simulink library "groundStation001_cl"  (R2018b)
settings: Solver=VariableStepAuto  StartTime=0.0  StopTime=10.0  RelTol=1e-3
undefined symbols (not defined in the file): CB2CMVec, flow, gndStnMmtArms, grav, inertiaMatrix, m, tetherLengths
libraries: thrAttachPtKinematics_ul x3, tethersMoment_cl x2, vrlib x1, eulAng2RotMat_ul x1, liftingBodyTension x1, circulationForce_ul x1, sixDoFDynamics_ul x1, tethers_cl x1, variableBuoyancy_ul x1
settings Model: Creator=Erin B  LastModifiedBy=mcobb

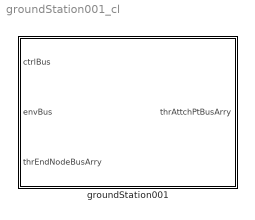
== system groundStation001_cl ==
  groundStation001 : Subsystem  mask{data=1, moments=0}
      mask prompts: data "Input lifting body forces or previously calculated lifting body forces? (0= input, 1 = previously calculated)"; moments "Calculate moments? (1 = yes, 0 = no)"

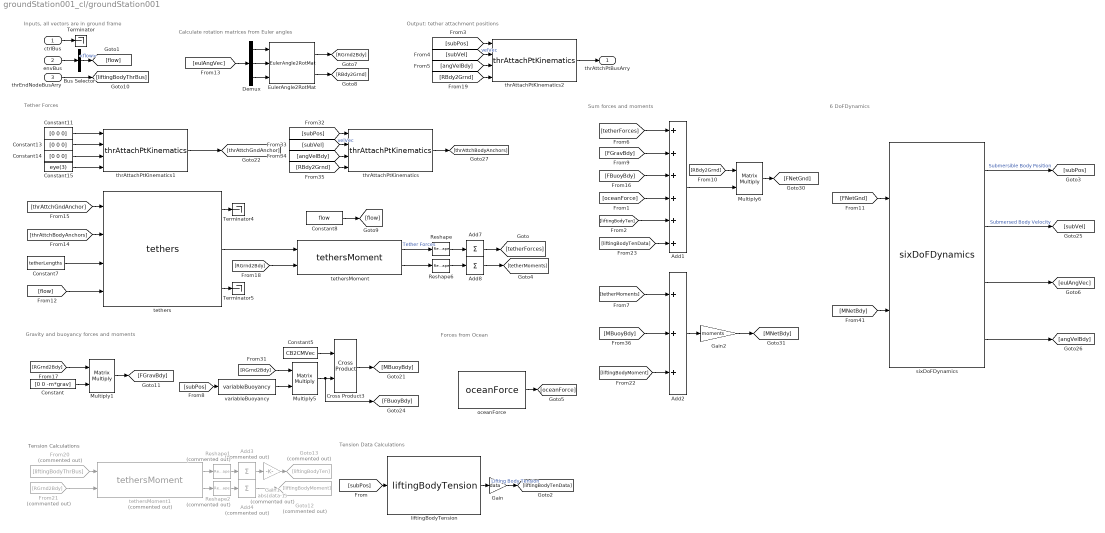
== system groundStation001_cl/groundStation001 ==
  note: Tension Calculations
  note: Tension Data Calculations
  note: Output: tether attachment positions
  note: Tether Forces
  note: Inputs, all vectors are in ground frame
  note: Calculate rotation matrices from Euler angles
  note: Sum forces and moments
  note: Gravity and buoyancy forces and moments
  note: 6 DoFDynamics
  note: Forces from Ocean
  ctrlBus : Inport  OutDataTypeStr=Bus: ctrlBus
  envBus : Inport  Port=2  OutDataTypeStr=Bus: envBus
  thrEndNodeBusArry : Inport  Port=3
  Add1 : Sum  Inputs=++++++
  Add2 : Sum  Inputs=+++
  Add3 : Sum  Commented=on  Inputs=+  CollapseMode=Specified dimension  CollapseDim=2
  Add4 : Sum  Commented=on  Inputs=+  CollapseMode=Specified dimension  CollapseDim=2
  Add7 : Sum  Inputs=+  CollapseMode=Specified dimension  CollapseDim=2
  Add8 : Sum  Inputs=+  CollapseMode=Specified dimension  CollapseDim=2
  Bus Selector : BusSelector  OutputSignals=flow
  Constant : Constant  Value=[0 0 -m*grav]
  Constant11 : Constant  Value=[0 0 0]
  Constant13 : Constant  Value=[0 0 0]
  Constant14 : Constant  Value=[0 0 0]
  Constant15 : Constant  Value=eye(3)
  Constant5 : Constant  Value=CB2CMVec
  Constant7 : Constant  Value=tetherLengths
  Constant8 : Constant  Value=flow
  Cross Product3 : vrlib/Utilities/Cross Product
      settings: SourceProductBaseCode=VR
  Demux : Demux  Outputs=3
  EulerAngle2RotMat : eulAng2RotMat_ul/EulerAngle2RotMat  SystemSampleTime=-1
  From20 : From  Commented=on  GotoTag=liftingBodyThrBus
  From21 : From  Commented=on  GotoTag=RGrnd2Bdy
  Gain : Gain  Gain=data
  Gain1 : Gain  Commented=on  Gain=abs(data-1)
  Gain2 : Gain  Gain=moments
  Goto12 : Goto  Commented=on  GotoTag=liftingBodyMoment
  Goto13 : Goto  Commented=on  GotoTag=liftingBodyTen
  Multiply1 : Product  Multiplication=Matrix(*)
  Multiply5 : Product  Multiplication=Matrix(*)
  Multiply6 : Product  Multiplication=Matrix(*)
  Reshape : Reshape  OutputDimensionality=Customize  OutputDimensions=[3 numel(gndStnMmtArms)]
  Reshape1 : Reshape  Commented=on  OutputDimensionality=Customize  OutputDimensions=[3 numel(gndStnMmtArms)]
  Reshape2 : Reshape  Commented=on  OutputDimensionality=Customize  OutputDimensions=[3 numel(gndStnMmtArms)]
  Reshape6 : Reshape  OutputDimensionality=Customize  OutputDimensions=[3 numel(gndStnMmtArms)]
  Terminator : Terminator
  Terminator4 : Terminator
  Terminator5 : Terminator
  liftingBodyTension : liftingBodyTension/liftingBodyTension  pos=position  mag=mag
  oceanForce : circulationForce_ul/oceanForce  SystemSampleTime=-1
  sixDoFDynamics : sixDoFDynamics_ul/sixDoFDynamics  M=mass  initPos=initPos  initVel=initVel  J=inertiaMatrix  initEulAngs=initEulerAngles  initAngVel=initAngVel
  tethers : tethers_cl/tethers   SystemSampleTime=-1
      link override VariantSubsystem: LabelModeActiveChoice=VSS_twoNodeTether
  tethersMoment : tethersMoment_cl/tethersMoment  arms=arms
  tethersMoment1 : tethersMoment_cl/tethersMoment  Commented=on  arms=arms
  thrAttachPtKinematics : thrAttachPtKinematics_ul/thrAttachPtKinematics  atchPts=bodyMmtArms
  thrAttachPtKinematics1 : thrAttachPtKinematics_ul/thrAttachPtKinematics  atchPts=gndStnMmtArms
  thrAttachPtKinematics2 : thrAttachPtKinematics_ul/thrAttachPtKinematics  atchPts=liftingBodyThrAttch
  variableBuoyancy : variableBuoyancy_ul/variableBuoyancy  vol=vol  h=h  grav=grav  rho=rho  waveAmplitude=waveAmp  oceanDepth=oceanDepth  wavePeriod=wavePeriod
  thrAttchPtBusArry : Outport
  wires:
  [RBdy2Grnd] -> Multiply6/1
  EulerAngle2RotMat/2 -> [RBdy2Grnd]
  sixDoFDynamics/4 -> [angVelBdy]
  variableBuoyancy/1 -> Multiply5/2
  [MBuoyBdy] -> Add2/2
  [tetherMoments] -> Add2/1
  [liftingBodyTen] -> Add1/5
  [FGravBdy] -> Add1/2
  [FBuoyBdy] -> Add1/3
  [FNetGnd] -> sixDoFDynamics/1
  tethers/3 -> Terminator5/1
  [thrAttchGndAnchor] -> tethers/1
  Add1/1 -> Multiply6/2
  Demux/2 -> EulerAngle2RotMat/2
  sixDoFDynamics/2 -> [subVel]  "Submersed Body Velocity"
  [flow] -> tethers/4
  [RGrnd2Bdy] -> Multiply5/1
  tethers/2 -> tethersMoment/1
  Cross Product3/1 -> [MBuoyBdy]
  tethers/1 -> Terminator4/1
  sixDoFDynamics/3 -> [eulAngVec]
  Multiply1/1 -> [FGravBdy]
  Multiply5/1 -> Cross Product3/2, [FBuoyBdy]
  Constant/1 -> Multiply1/2
  [thrAttchBodyAnchors] -> tethers/2
  sixDoFDynamics/1 -> [subPos]  "Submersible Body Position"
  Multiply6/1 -> [FNetGnd]
  [RGrnd2Bdy] -> tethersMoment/2
  Demux/1 -> EulerAngle2RotMat/1
  Constant5/1 -> Cross Product3/1
  [eulAngVec] -> Demux/1
  Demux/3 -> EulerAngle2RotMat/3
  [RGrnd2Bdy] -> Multiply1/1
  [tetherForces] -> Add1/1
  EulerAngle2RotMat/1 -> [RGrnd2Bdy]
  Constant7/1 -> tethers/3
  [MNetBdy] -> sixDoFDynamics/2
  Constant8/1 -> [flow]
  [subPos] -> variableBuoyancy/1
  [subPos] -> thrAttachPtKinematics/1
  [angVelBdy] -> thrAttachPtKinematics/3
  [RBdy2Grnd] -> thrAttachPtKinematics/4
  thrAttachPtKinematics/1 -> [thrAttchBodyAnchors]
  [subVel] -> thrAttachPtKinematics/2  "velVec"
  Constant11/1 -> thrAttachPtKinematics1/1
  Constant13/1 -> thrAttachPtKinematics1/2
  Constant14/1 -> thrAttachPtKinematics1/3
  Constant15/1 -> thrAttachPtKinematics1/4
  thrAttachPtKinematics1/1 -> [thrAttchGndAnchor]
  tethersMoment/1 -> Reshape/1  "Tether Forces"
  Reshape/1 -> Add7/1
  tethersMoment/2 -> Reshape6/1
  Reshape6/1 -> Add8/1
  Add7/1 -> [tetherForces]
  Add8/1 -> [tetherMoments]
  oceanForce/1 -> [oceanForce]
  [oceanForce] -> Add1/4
  [subVel] -> thrAttachPtKinematics2/2  "velVec"
  [RBdy2Grnd] -> thrAttachPtKinematics2/4
  [angVelBdy] -> thrAttachPtKinematics2/3
  [subPos] -> thrAttachPtKinematics2/1
  thrAttachPtKinematics2/1 -> thrAttchPtBusArry/1
  [subPos] -> liftingBodyTension/1
  thrEndNodeBusArry/1 -> [liftingBodyThrBus]
  From20/1 -> tethersMoment1/1
  From21/1 -> tethersMoment1/2
  Reshape1/1 -> Add3/1
  Reshape2/1 -> Add4/1
  Add4/1 -> Goto12/1
  tethersMoment1/1 -> Reshape1/1
  tethersMoment1/2 -> Reshape2/1
  [liftingBodyMoment] -> Add2/3
  Gain/1 -> [liftingBodyTenData]  "Lifting Body Tension"
  liftingBodyTension/1 -> Gain/1
  [liftingBodyTenData] -> Add1/6
  Add3/1 -> Gain1/1
  Gain1/1 -> Goto13/1
  Add2/1 -> Gain2/1
  Gain2/1 -> [MNetBdy]
  envBus/1 -> Bus Selector/1
  ctrlBus/1 -> Terminator/1
  Bus Selector/1 -> [flow]  "<flow>"
